simulink model "Final_Q2_F"  (R2019a)
settings: Solver=ode1  StartTime=0.0  StopTime=60  FixedStep=0.01  RelTol=1e-3  EnableMultiTasking=on
settings Model: Creator=enesu  LastModifiedBy=hp
settings SolverCC: AutoInsertRateTranBlk=on

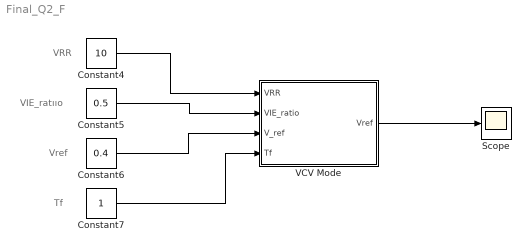
== system Final_Q2_F ==
  note: Tf
  note: Vref
  note: VIE_ratııo
  note: VRR
  Constant4 : Constant  Value=10
  Constant5 : Constant  Value=0.5
  Constant6 : Constant  Value=0.4
  Constant7 : Constant
  Scope : Scope
  VCV Mode : Subsystem
  wires:
  Constant6/1 -> VCV Mode/3(V_ref)
  Constant5/1 -> VCV Mode/2(VIE_ratio)
  Constant4/1 -> VCV Mode/1(VRR)
  Constant7/1 -> VCV Mode/4(Tf)
  VCV Mode/1("Vref ") -> Scope/1

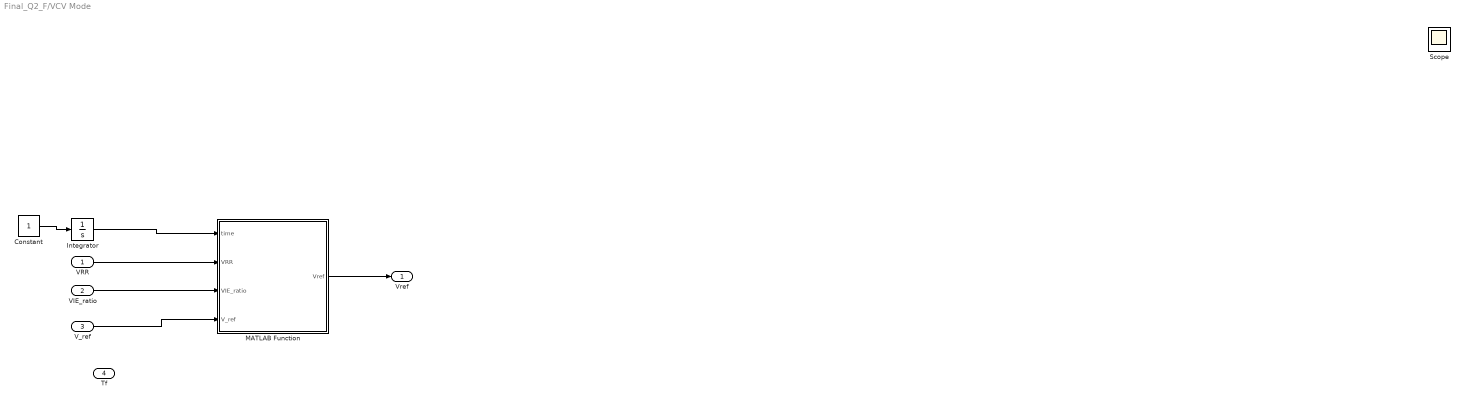
== system Final_Q2_F/VCV Mode ==
  VRR : Inport
  VIE_ratio : Inport  Port=2
  V_ref : Inport  Port=3
  Tf : Inport  Port=4
  Constant : Constant
  Integrator : Integrator
  MATLAB Function : MATLAB Function  TreatAsAtomicUnit=on
  Scope : Scope  NumInputPorts=3
  "Vref " : Outport  VectorParamsAs1DForOutWhenUnconnected=on
  wires:
  Constant/1 -> Integrator/1
  Integrator/1 -> MATLAB Function/1(time)
  VRR/1 -> MATLAB Function/2(VRR)
  VIE_ratio/1 -> MATLAB Function/3(VIE_ratio)
  V_ref/1 -> MATLAB Function/4(V_ref)
  MATLAB Function/1(Vref) -> "Vref "/1

== matlab function Final_Q2_F/VCV Mode/MATLAB Function ==
  data: time input; Vref output; VRR input; VIE_ratio input; V_ref input
function Vref = Vref_producer(time,VRR,VIE_ratio ,V_ref)

stop_time = 60; % stop time is given as 60 seconds

% Ti - Inspiratory Time (s)     Te - Expiratory Time (s)
% VRR - Ventilator Respiratory Rate (breaths/min) is 10.
% VIE_ratio ventilator inspiratory/expiratory rate is 0.5.
% 
% There are 2 two equations.
%
%   60
% ------ = Ti + Te     and     Ti = Te x VIE_ratio
%   VRR
% 
% in matrix form;
%  _  _     _             _     _  _
% | 60 |   | 1      1      |   | Ti |
% | 0  | = | 1  -VIE_ratio | * | Te |
%  -  -     -             -     -  -
%
%   b = A.T 
%   T = inv(A).b

A = [ 1 1 ; 1 -VIE_ratio];
B = [stop_time/VRR ; 0];

T = inv(A)*B;

Ti = T(1); % Ti
Te = T(2); % Te



% We can set the period duration of the desired square wave 
% as [0, Ti + Te] by performing modulus operation.
time = mod(time , Ti + Te ); 

if( time <= Ti)
    Vref = V_ref; 
else
    Vref = 0; 
end
end
